simulink library "MIL_Test"  (Simulink 6.6)
undefined symbols (not defined in the file or in its folder): getdatatypespecs, slcm, StepSize
libraries: simulink x71, MIL_Test x6
(part 3 of 8)

== system MIL_Test/Validation Function/Feature extraction/Complete step detection/Step detection ==
  R : Inport
  Step : Inport  Port=2
  Step response : Inport  Port=3
  Active if signals constant for some specified time : Subsystem
  Detect constant : Subsystem  TreatAsAtomicUnit=on  mask(Feature extraction block){RT=0.0001}
      mask prompts: RT "Relative tolerance in %"
      mask help: Detect if the signal value is constant (using the last two signal values) allowing for a user-defined relative deviation
      mask CallbackString:
      | if or( (str2double(get_param(gcb,'RT')) < 0), (str2double(get_param(gcb,'RT')) > 100))
      |     error(['Relative tolerance value (' get_param(gcb,'RT') ') out of range. Please give a value between 0 and 100.']);
      | else
      |     set_param([gcb '/Relative tolerance/Relative Tolerance'],'Value',get_param(gcb,'RT'));
      | end
  Detect decrease : Subsystem  TreatAsAtomicUnit=on  mask(Detect increase){Param=0}
      mask prompts: Param "Mask Parameter 1:"
  Detect increase : Subsystem  TreatAsAtomicUnit=on  mask(Detect increase){Param=0}
      mask prompts: Param "Mask Parameter 1:"
  Detect increase2 : Subsystem  TreatAsAtomicUnit=on  mask(Detect increase){Param=0}
      mask prompts: Param "Mask Parameter 1:"
  Hold1 : Subsystem  TreatAsAtomicUnit=on
      mask Display: patch(-0.31+[0.4 0.46 0.46 0.54 0.54 0.6 0.6 0.55 0.55 0.45 0.45 0.4],-0.19+[0.85 0.85 0.95 0.95 0.85 0.85 0.87 0.87 0.96 0.96 0.87 0.87],[0 0 0]);
  Logical Operator : Logic  AllPortsSameDT=off  OutDataTypeMode=Boolean
  Logical Operator1 : Logic  Operator=NOT  AllPortsSameDT=off  OutDataTypeMode=Boolean
  Logical Operator2 : Logic  Operator=OR  Inputs=3  AllPortsSameDT=off  OutDataTypeMode=Boolean
  Memory2 : Memory
  End of complete step : Outport
  wires:
  Detect increase/1(Increase) -> Logical Operator2/1
  Detect constant/1(Constant) -> Logical Operator1/1
  Detect decrease/1(Decrease) -> Logical Operator2/2
  Logical Operator2/1 -> Hold1/1(" ")
  R/1 -> Hold1/2("    ")
  Step/1 -> Active if signals constant for some specified time/1(Signal1), Detect constant/1(Signal)
  Step response/1 -> Active if signals constant for some specified time/2(Signal 2)
  Active if signals constant for some specified time/1(Constant signals) -> Detect decrease/1(Signal), Detect increase/1(Signal), Detect increase2/1(Signal)
  Hold1/1("  ") -> Memory2/1
  Logical Operator/1 -> End of complete step/1
  Memory2/1 -> Logical Operator/2
  Detect increase2/1(Increase) -> Logical Operator/1
  Logical Operator1/1 -> Logical Operator2/3

== system MIL_Test/Validation Function/Feature extraction/Complete step detection/Step detection reset ==
  Step : Inport
  Step response : Inport  Port=2
  Active if signals constant for some specified time : Subsystem
  Logical Operator : Logic  AllPortsSameDT=off  OutDataTypeMode=Boolean
  Memory : Memory
  Step detection : Subsystem  TreatAsAtomicUnit=on  mask(Feature extraction block){StepSize=10}
      mask prompts: StepSize "Minimum step size"
      mask help: Detect a step in the signal. The minimum step size is defined by the user.
      mask CallbackString:
      | if str2double(get_param(gcb,'StepSize')) <= 0
      |     error(['Minimum step size (' get_param(gcb,'StepSize') ') out of range. Please give a value greater than zero.']);
      | else
      |     set_param([gcb '/Min step size'],'Value',get_param(gcb,'StepSize'));
      | end
  R : Outport
  wires:
  Logical Operator/1 -> R/1
  Step detection/1(Step) -> Logical Operator/2
  Step response/1 -> Active if signals constant for some specified time/1(Signal1)
  Memory/1 -> Logical Operator/1
  Active if signals constant for some specified time/1(Constant signals) -> Memory/1
  Step/1 -> Active if signals constant for some specified time/2(Signal 2), Step detection/1(Signal)

== system MIL_Test/Validation Function/Feature extraction/Detect constant/Relative tolerance ==
  sig : Inport
  ref : Inport  Port=2
  Abs : Abs
  Abs1 : Abs
  Add : Sum  Inputs=+-  OutScaling=2^-10
  Divide1 : Product  Inputs=**/  OutScaling=2^-10
  Max : Constant  Value=100
  Relational Operator : RelationalOperator  Operator===  LogicOutDataTypeMode=Boolean
  Relative Tolerance : Constant
  sig == ref : Outport
  wires:
  Abs1/1 -> Divide1/1
  Relational Operator/1 -> sig == ref/1
  Relative Tolerance/1 -> Divide1/2
  Max/1 -> Divide1/3
  Divide1/1 -> Relational Operator/2
  ref/1 -> Abs1/1, Add/2
  sig/1 -> Add/1
  Add/1 -> Abs/1
  Abs/1 -> Relational Operator/1

== system MIL_Test/Validation Function/Feature extraction/Linear relation/Relative tolerance ==
  sig : Inport
  ref : Inport  Port=2
  Abs : Abs
  Abs1 : Abs
  Add : Sum  Inputs=+-  OutScaling=2^-10
  Divide1 : Product  Inputs=**/  OutScaling=2^-10
  Max : Constant  Value=100
  Relational Operator : RelationalOperator  Operator=<=  LogicOutDataTypeMode=Boolean
  Relative Tolerance : Constant  Value=0.0001
  sig == ref : Outport
  wires:
  Abs1/1 -> Divide1/1
  Relational Operator/1 -> sig == ref/1
  Relative Tolerance/1 -> Divide1/2
  Max/1 -> Divide1/3
  Divide1/1 -> Relational Operator/2
  ref/1 -> Abs1/1, Add/2
  sig/1 -> Add/1
  Add/1 -> Abs/1
  Abs/1 -> Relational Operator/1

== system MIL_Test/Validation Function/Feature extraction/Signal value @ maximum/Local maximum ==
  Signal : Inport
  Clock : Clock
      settings: Decimation=10
  Clock1 : Clock
      settings: Decimation=10
  Logical Operator : Logic  AllPortsSameDT=off  OutDataTypeMode=Boolean
  Memory : Memory
  Memory1 : Memory
  Relational Operator : RelationalOperator  Operator=<  LogicOutDataTypeMode=Boolean
  Relational Operator1 : RelationalOperator  Operator=>  LogicOutDataTypeMode=Boolean
  Switch : Switch  Criteria=u2 > Threshold
  Switch1 : Switch  Criteria=u2 > Threshold
  Maximum : Outport
  wires:
  Switch1/1 -> Relational Operator1/2
  Memory1/1 -> Switch1/1
  Clock1/1 -> Switch1/2
  Switch/1 -> Relational Operator1/1, Switch1/3, Memory1/1, Relational Operator/2
  Memory/1 -> Switch/1
  Clock/1 -> Switch/2
  Relational Operator/1 -> Logical Operator/1
  Relational Operator1/1 -> Logical Operator/2
  Logical Operator/1 -> Maximum/1
  Signal/1 -> Switch/3, Memory/1, Relational Operator/1

== system MIL_Test/Validation Function/Feature extraction/Step response characteristics/Step response characteristics extraction ==
  R : Inport
  Step : Inport  Port=2
  Step response : Inport  Port=3
  Clock : Clock
      settings: Decimation=10
  Expected set point and step parameters : Subsystem  TreatAsAtomicUnit=on
  Extract maximum overshoot : Subsystem
  Extract rise time : Subsystem
  Extract settling time : Subsystem
  Extract steady state error : Subsystem
  Memory : Memory
  Static Gain : Constant  Value=0.8333
  Step time : Subsystem  TreatAsAtomicUnit=on
  Rise time : Outport  DataType=double
  Maximum overshoot : Outport  Port=2  DataType=double
  Settling time : Outport  Port=3  DataType=double
  Steady state error : Outport  Port=4  DataType=double
  wires:
  Expected set point and step parameters/1(Step sign) -> Extract maximum overshoot/3(Step sign)
  Expected set point and step parameters/3(Response step size) -> Extract rise time/4(Response step size)
  Step response/1 -> Extract rise time/1(Step response), Extract maximum overshoot/1(Step response), Extract settling time/1(Step response), Extract steady state error/1(Step response)
  Step time/1(Time) -> Extract settling time/4(Step time)
  Expected set point and step parameters/2(Set point) -> Extract rise time/3(Set point), Extract settling time/2(Set point), Extract steady state error/2(Set point)
  Extract steady state error/1(ss error) -> Steady state error/1
  Memory/1 -> Expected set point and step parameters/1(Step/z)
  Clock/1 -> Step time/1(Clock)
  Step/1 -> Expected set point and step parameters/2(Step), Memory/1
  R/1 -> Extract settling time/3(Reset), Extract maximum overshoot/2(Reset), Extract rise time/2(Reset), Expected set point and step parameters/Trigger, Step time/Trigger
  Static Gain/1 -> Expected set point and step parameters/3(Static Gain)
  Extract settling time/1(Settling time) -> Settling time/1
  Extract maximum overshoot/1(Maximum overshoot) -> Maximum overshoot/1
  Extract rise time/1(Rise time) -> Rise time/1

== system MIL_Test/Validation Function/Feature extraction/Step response characteristics/Step response reset ==
  Step : Inport
  Step response : Inport  Port=2
  Active if signals constant for some specified time : Subsystem
  Logical Operator : Logic  AllPortsSameDT=off  OutDataTypeMode=Boolean
  Memory : Memory
  Step detection : Subsystem  TreatAsAtomicUnit=on  mask(Feature extraction block){StepSize=1}
      mask prompts: StepSize "Minimum step size"
      mask help: Detect a step in the signal. The minimum step size is defined by the user.
      mask CallbackString:
      | if str2double(get_param(gcb,'StepSize')) <= 0
      |     error(['Minimum step size (' get_param(gcb,'StepSize') ') out of range. Please give a value greater than zero.']);
      | else
      |     set_param([gcb '/Min step size'],'Value',get_param(gcb,'StepSize'));
      | end
  R : Outport
  wires:
  Logical Operator/1 -> R/1
  Step detection/1(Step) -> Logical Operator/2
  Step response/1 -> Active if signals constant for some specified time/1(Signal1)
  Memory/1 -> Logical Operator/1
  Active if signals constant for some specified time/1(Constant signals) -> Memory/1
  Step/1 -> Active if signals constant for some specified time/2(Signal 2), Step detection/1(Signal)

== system MIL_Test/Validation Function/Feature extraction/Step response characteristics/Step response trigger ==
  Steady state error : Inport
  Step response : Inport  Port=2
  Abs : Abs
  Active if signals constant for some specified time : Subsystem
  Compare To Constant : Subsystem  mask(Compare To Constant){relop=<=, const=0.5, LogicOutDataTypeMode=uint8, ZeroCross=off}
      mask prompts: relop "Operator:"; const "Constant value:"; LogicOutDataTypeMode "Output data type mode:"; ZeroCross "Enable zero crossing detection"
      mask help: Determine how a signal compares to a constant.
      mask init:
      | blkName = gcb;
      | 
      | if strcmp(get_param(gcbh,'LogicOutDataTypeMode'),'boolean')
      | 	setValue = 'Boolean';
      | else
      | 	setValue = 'Specify via dialog';
      | end
      | 
      | set_param([blkName,'/Compare'],'relop',relop, ...
      | 	'LogicOutDataTypeMode', setValue, 'ZeroCross', ZeroCross);
      | 
      | if length(const) == 1
      |  str = [relop,' ',num2str(double(const))];
      | else
      |   str = [relop,' C'];
      | end
      mask StyleString: popup(==|~=|<|<=|>=|>),edit,popup(uint8|boolean),checkbox
      mask Display: disp(str)
  Data Type Conversion : DataTypeConversion
  Data Type Conversion1 : DataTypeConversion
  Detect increase : Subsystem  TreatAsAtomicUnit=on
  Logical Operator : Logic  AllPortsSameDT=off  OutDataTypeMode=Boolean  LogicDataType=double
  Rise time T : Outport  DataType=double
  Overshoot T : Outport  Port=2  DataType=double
  Settling time T : Outport  Port=3  DataType=double
  Steady state error T : Outport  Port=4  DataType=double
  wires:
  Logical Operator/1 -> Data Type Conversion/1
  Detect increase/1(Increase) -> Data Type Conversion1/1, Logical Operator/2
  Abs/1 -> Compare To Constant/1(u)
  Compare To Constant/1(y) -> Logical Operator/1
  Steady state error/1 -> Abs/1
  Step response/1 -> Active if signals constant for some specified time/1(Signal1), Active if signals constant for some specified time/2(Signal 2)
  Active if signals constant for some specified time/1(Constant signals) -> Detect increase/1(Signal)
  Data Type Conversion1/1 -> Steady state error T/1
  Data Type Conversion/1 -> Settling time T/1, Overshoot T/1, Rise time T/1

== system MIL_Test/Validation Function/Feature extraction/Time @ sig = x/Relative tolerance ==
  sig : Inport
  ref : Inport  Port=2
  Abs : Abs
  Abs1 : Abs
  Add : Sum  Inputs=+-  OutScaling=2^-10
  Divide1 : Product  Inputs=**/  OutScaling=2^-10
  Max : Constant  Value=100
  Relational Operator : RelationalOperator  Operator=<=  LogicOutDataTypeMode=Boolean
  Relative Tolerance : Constant  Value=0.0001
  sig == ref : Outport
  wires:
  Abs1/1 -> Divide1/1
  Relational Operator/1 -> sig == ref/1
  Relative Tolerance/1 -> Divide1/2
  Max/1 -> Divide1/3
  Divide1/1 -> Relational Operator/2
  ref/1 -> Abs1/1, Add/2
  sig/1 -> Add/1
  Add/1 -> Abs/1
  Abs/1 -> Relational Operator/1

== system MIL_Test/Validation Function/Feature extraction/Time since signal constant/Detect constant ==
  Signal : Inport
  Clock : Clock
      settings: Decimation=10
  Constant1 : Constant  Value=0  OutDataTypeMode=boolean
  Memory : Memory
  Relative tolerance : Subsystem
  Switch : Switch  Criteria=u2 > Threshold
  Constant : Outport
  wires:
  Switch/1 -> Constant/1
  Relative tolerance/1(sig == ref) -> Switch/1
  Clock/1 -> Switch/2
  Constant1/1 -> Switch/3
  Memory/1 -> Relative tolerance/2(ref)
  Signal/1 -> Relative tolerance/1(sig), Memory/1

== system MIL_Test/Validation Function/TODO/<system name>/<Requirement name> ==
  InOut Bus : Inport
  <Assertions name> : Subsystem  Description=Assertions template. Create a new assertions block from this template.
  <Preconditions name> : Subsystem  Description=Preconditions template. Create new preconditions blocks using this template.
  Bus Creator : BusCreator  Inputs=1
  Test Info : Outport
  wires:
  <Preconditions name>/1(Activate) -> <Assertions name>/1(Precond)
  Bus Creator/1 -> Test Info/1
  <Assertions name>/1(VF info) -> Bus Creator/1
  InOut Bus/1 -> <Preconditions name>/1(InOut Bus), <Assertions name>/2(InOut Bus)

== system MIL_Test/Validation Function/TODO/Assertions/Fault info ==
  Local Verdict : Inport
  Expected lower limit : Inport  Port=2
  Expected upper limit : Inport  Port=3
  Actual Data : Inport  Port=4
  Enable : EnablePort
  Assertions : Constant  Value=Ass
  Bus Creator : BusCreator  Inputs=5
  Bus Creator1 : BusCreator  Inputs=3
  Data Type Conversion{,1..3} (4 alike) : DataTypeConversion
  Preconditions : Constant  Value=Pre
  Requirement : Constant  Value=Req
  VF info : Outport  OutputWhenDisabled=reset  InitialOutput=[2]
  wires:
  Requirement/1 -> Bus Creator1/3  "Requirement"
  Preconditions/1 -> Bus Creator1/2  "Preconditions"
  Assertions/1 -> Bus Creator1/1  "Assertions"
  Data Type Conversion3/1 -> Bus Creator/4  "Actual data"
  Data Type Conversion2/1 -> Bus Creator/3  "Expected upper limit"
  Data Type Conversion1/1 -> Bus Creator/2  "Expected lower limit"
  Data Type Conversion/1 -> Bus Creator/1  "Local verdict"
  Local Verdict/1 -> Data Type Conversion/1  "Local verdict"
  Expected upper limit/1 -> Data Type Conversion2/1  "Expected upper limit"
  Expected lower limit/1 -> Data Type Conversion1/1  "Expected lower limit"
  Actual Data/1 -> Data Type Conversion3/1  "Actual Data"
  Bus Creator1/1 -> Bus Creator/5  "Source"
  Bus Creator/1 -> VF info/1

== system MIL_Test/Validation Function/TODO/Assertions/Signal comparison ==
  Bound : Subsystem  mask(Bound){cm=>=, Lower=0, Upper=1}
      mask prompts: cm "Comparison method:"; Upper "Mask Parameter 3:"
      mask help:
      | Compare a signal with a reference using the specified comparison method.
      |
      | Output verdict V and lower (LL) and upper (UL) limits for reporting.
      |
      | For '==' or '~=' use "Range - Gap"
      mask init:
      | set_param([get_param(gcb,'Parent') '/' get_param(gcb,'Name') '/Relational Operator'],'Operator',get_param(gcb,'cm'));
      | set_param(gcb,'Upper',num2str(uint8(max(get_param([get_param(gcb,'Parent') '/' get_param(gcb,'Name') '/Relational Operator'],'Operator') == '>'))));
      | set_param(gcb,'Lower',num2str(uint8(max(get_param([get_param(gcb,'Parent') '/' get_param(gcb,'Name') '/Relational Operator'],'Operator') == '<'))));
      mask StyleString: popup(>|>=|<=|<),edit,edit
      mask Display:
      | port_label('output', 1, 'V');
      | port_label('output', 2, 'LL');
      | port_label('output', 3, 'UL');
      | port_label('input', 1, 'Sig');
      | port_label('input', 2, 'Ref');
      | text(0.05,0.5,get_param(get_param([get_param(gcb,'Parent') '/' get_param(gcb,'Name') '/Relational Operator'],'handle'),'Operator'));
  Range - Gap Absolute tolerance : Subsystem  mask(Range - Gap Absolute Tolerance){GorR=Range, AbsoluteTolerance=100}
      mask prompts: GorR "Use range or gap"; AbsoluteTolerance "Absolute Tolerance"
      mask help:
      | Check that a signal stays inside a range or outside a gap around a reference signal. Specify the range or the gap absolute to the reference signal.
      |
      | Output verdict V and lower (LL) and upper (UL) limits for reporting.
      mask init: same as MIL_Test/Test Data/Signal comparison/Range - Gap Relative tolerance Precond
      mask StyleString: popup(Range|Gap  ),edit
      mask Display:
      | port_label('output',1,'V');
      | port_label('output',2,'LL');
      | port_label('output',3,'UL');
      | port_label('input',1,'Sig');
      | port_label('input',2,'Ref');
      | text(0.40,0.53,'+');
      | text(0.415,0.46,'-');
      | text(0.5,0.5,num2str(AbsoluteTolerance));
      | text(0.05,0.5,helpVariable2);
  Range - Gap Relative tolerance : Subsystem  mask(Range - Gap Relative Tolerance){GorR=Range, RelativeTolerance=1}
      mask prompts: GorR "Use range or gap"; RelativeTolerance "Relative Tolerance in Percent"
      mask help:
      | Check that a signal stays inside a range or outside a gap around a reference signal. Specify the range or the gap relative to the reference signal.
      |
      | Output verdict V and lower (LL) and upper (UL) limits for reporting.
      mask init: same as MIL_Test/Test Data/Signal comparison/Range - Gap Relative tolerance Precond
      mask StyleString: popup(Range|Gap  ),edit
      mask Display:
      | port_label('output',1,'V');
      | port_label('output',2,'LL');
      | port_label('output',3,'UL');
      | port_label('input',1,'Sig');
      | port_label('input',2,'Ref');
      | text(0.425,0.5,[num2str(RelativeTolerance) ' %']);
      | text(0.05,0.5,helpVariable2);
  Range - Gap Tolerance range : Subsystem  mask(Range - Gap Tolerance range){GorR=Range}
      mask prompts: GorR "Use range or gap"
      mask help:
      | Check that a signal stays inside a dynamically specified value range.
      |
      | Output verdict V and lower (LL) and upper (UL) limits for reporting.
      mask init:
      | if max(get_param(gcb,'GorR') == ' ') % Gap
      |     helpVariable1 = '<=';
      | else % Range
      |     helpVariable1 = '>=';
      | end
      | set_param([get_param(gcb,'Parent') '/' get_param(gcb,'Name') '/Relational Operator'],'Operator',helpVariable1);
      | clear helpVariable1;
      mask StyleString: popup(Range|Gap  )
      mask Display:
      | port_label('output',1,'V');
      | port_label('output',2,'LL');
      | port_label('output',3,'UL');
      | port_label('input',1,'Sig');
      | port_label('input',2,'Lower Bound');
      | port_label('input',3,'Upper Bound');
      | patch(0.05+[0.3 0.7 0.7 0.3],-0.05+[0.8 0.8 0.9 0.9],[1 1 1]*double(not(max(get_param(gcb,'GorR') == ' '))));
      | patch(0.05+[0.3 0.7 0.7 0.3],-0.05+[0.9 0.9 0.95 0.95],[1 1 1]*double(max(get_param(gcb,'GorR') == ' ')));
      | patch(0.05+[0.3 0.7 0.7 0.3],-0.05+[0.75 0.75 0.8 0.8],[1 1 1]*double(max(get_param(gcb,'GorR') == ' ')));
      | patch(0.05+[0.25 0.25 0.8 0.8 0.26 0.26],[0.95 0.65 0.65 0.66 0.66 0.95],[0 0 0]);
      | patch(0.033+[0.27 0.22 0.23 0.27 0.31 0.32 0.27],0.02+[0.95 0.85 0.85 0.89 0.85 0.85 0.95],[0 0 0]);
      | patch(0.17+[0.7 0.6 0.6 0.65 0.6 0.6 0.7],-0.043+[0.7 0.63 0.64 0.7 0.76 0.77 0.7],[0 0 0]);

== system MIL_Test/Validation Function/TODO/Model Info/EmptySubsystem ==

== system MIL_Test/Validation Function/TODO/Preconditions/Signal comparison ==
  Bound : Subsystem  mask(Bound){cm=>=}
      mask prompts: cm "Comparison method:"
      mask help:
      | Compare a signal with a reference using the specified comparison method.
      |
      | For '==' or '~=' use "Range - Gap"
      mask init:
      | bp = get_param(gcbh,'Parent');
      | bn = get_param(gcbh,'Name');
      | set_param([bp '/' bn '/RelOp'],'Operator',get_param(gcbh,'cm'));
      mask StyleString: popup(>|>=|<=|<)
      mask Display:
      | port_label('output', 1, 'A');
      | port_label('input', 1, 'Sig');
      | port_label('input', 2, 'Ref');
      | text(0.05,0.5,get_param(get_param([get_param(gcb,'Parent') '/' get_param(gcb,'Name') '/RelOp'],'handle'),'Operator'));
  Range - Gap Absolute tolerance : Subsystem  mask(Range - Gap Absolute Tolerance){GorR=Range, AbsoluteTolerance=100}
      mask prompts: GorR "Use range or gap"; AbsoluteTolerance "Absolute Tolerance"
      mask help: Check that a signal stays inside a range or outside a gap around a reference signal. Specify the range or the gap absolute to the reference signal.
      mask init:
      | if max(get_param(gcb,'GorR') == ' ') % Gap
      |     helpVariable1 = '>=';
      |     helpVariable2 = '~=';
      | else % Range
      |     helpVariable1 = '<=';
      |     helpVariable2 = '==';
      | end
      | set_param([get_param(gcb,'Parent') '/' get_param(gcb,'Name') '/Relational Operator'],'Operator',helpVariable1);
      | set_param(gcb,'Op',helpVariable2);
      | clear helpVariable1;
      mask StyleString: popup(Range|Gap  ),edit
      mask Display:
      | port_label('output',1,'A');
      | port_label('input',1,'Sig');
      | port_label('input',2,'Ref');
      | text(0.40,0.53,'+');
      | text(0.415,0.46,'-');
      | text(0.5,0.5,num2str(AbsoluteTolerance));
      | text(0.05,0.5,helpVariable2);
  Range - Gap Relative tolerance : Subsystem  mask(Range - Gap Relative Tolerance){GorR=Range, RelativeTolerance=1}
      mask prompts: GorR "Use range or gap"; RelativeTolerance "Relative Tolerance in Percent"
      mask help: Check that a signal stays inside a range or outside a gap around a reference signal. Specify the range or the gap relative to the reference signal.
      mask init: same as MIL_Test/Test Data/Signal comparison/Range - Gap Relative tolerance Precond
      mask StyleString: popup(Range|Gap  ),edit
      mask Display:
      | port_label('output',1,'A');
      | port_label('input',1,'Sig');
      | port_label('input',2,'Ref');
      | text(0.425,0.5,[num2str(RelativeTolerance) ' %']);
      | text(0.05,0.5,helpVariable2);
  Range - Gap Tolerance range : Subsystem  mask(Range - Gap Tolerance range){GorR=Range}
      mask prompts: GorR "Use range or gap"
      mask help: Check that a signal stays inside a dynamically specified value range.
      mask init: same as MIL_Test/Validation Function/TODO/Assertions/Signal comparison/Range - Gap Tolerance range
      mask StyleString: popup(Range|Gap  )
      mask Display:
      | port_label('output',1,'A');
      | port_label('input',1,'Sig');
      | port_label('input',2,'Lower Bound');
      | port_label('input',3,'Upper Bound');
      | patch(0.05+[0.3 0.7 0.7 0.3],-0.05+[0.8 0.8 0.9 0.9],[1 1 1]*double(not(max(get_param(gcb,'GorR') == ' '))));
      | patch(0.05+[0.3 0.7 0.7 0.3],-0.05+[0.9 0.9 0.95 0.95],[1 1 1]*double(max(get_param(gcb,'GorR') == ' ')));
      | patch(0.05+[0.3 0.7 0.7 0.3],-0.05+[0.75 0.75 0.8 0.8],[1 1 1]*double(max(get_param(gcb,'GorR') == ' ')));
      | patch(0.05+[0.25 0.25 0.8 0.8 0.26 0.26],[0.95 0.65 0.65 0.66 0.66 0.95],[0 0 0]);
      | patch(0.033+[0.27 0.22 0.23 0.27 0.31 0.32 0.27],0.02+[0.95 0.85 0.85 0.89 0.85 0.85 0.95],[0 0 0]);
      | patch(0.17+[0.7 0.6 0.6 0.65 0.6 0.6 0.7],-0.043+[0.7 0.63 0.64 0.7 0.76 0.77 0.7],[0 0 0]);

== system MIL_Test/Validation Function/TODO/Validation FunctionsTemplate/Arbitration ==
  In1 : Inport
  Collect Verdicts : MinMax  Inputs=3
  Memory : Memory  Orientation=left  X0=2
  Out1 : Outport
  wires:
  Collect Verdicts/1 -> Memory/1, Out1/1
  In1/1 -> Collect Verdicts/1
  Memory/1 -> Collect Verdicts/3

== system MIL_Test/Validation Function/TODO/Validation FunctionsTemplate/Datatype conversion ==
  InOutBus : Inport
  Bus Creator{,1..5} (6 alike) : BusCreator  Inputs=2
  Bus Selector : BusSelector  OutputSignals=Inputs,Outputs
  Bus Selector1 : BusSelector  OutputSignals=v_Fzg,signal2
  Bus Selector2 : BusSelector  OutputSignals=signal1,signal2
  Bus Selector3 : BusSelector  OutputSignals=phi_Acc,phi_Brake
  Bus Selector4 : BusSelector  OutputSignals=T_des_Drive,T_des_Brake
  Bus Selector5 : BusSelector  OutputSignals=AccPedal,BrakePedal
  Data Type Conversion{,1..6} (7 alike) : DataTypeConversion
  InOut Bus : Outport
  wires:
  Bus Creator5/1 -> InOut Bus/1  "InOutBus"
  Bus Creator4/1 -> Bus Creator5/2  "Outputs"
  Bus Creator3/1 -> Bus Creator5/1  "Inputs"
  Bus Creator1/1 -> Bus Creator4/2
  Bus Creator/1 -> Bus Creator4/1
  Data Type Conversion/1 -> Bus Creator3/1  "v_Fzg"
  Bus Creator2/1 -> Bus Creator3/2  "signal2"
  Data Type Conversion2/1 -> Bus Creator2/2  "phi_Brake"
  Data Type Conversion1/1 -> Bus Creator2/1  "phi_Acc"
  Data Type Conversion6/1 -> Bus Creator1/2  "BrakePedal"
  Data Type Conversion5/1 -> Bus Creator1/1  "AccPedal"
  Data Type Conversion4/1 -> Bus Creator/2  "T_des_Brake"
  Data Type Conversion3/1 -> Bus Creator/1  "T_des_Drive"
  Bus Selector5/2 -> Data Type Conversion6/1  "<BrakePedal>"
  Bus Selector5/1 -> Data Type Conversion5/1  "<AccPedal>"
  Bus Selector4/2 -> Data Type Conversion4/1  "<T_des_Brake>"
  Bus Selector4/1 -> Data Type Conversion3/1  "<T_des_Drive>"
  Bus Selector3/2 -> Data Type Conversion2/1  "<phi_Brake>"
  Bus Selector3/1 -> Data Type Conversion1/1  "<phi_Acc>"
  Bus Selector1/1 -> Data Type Conversion/1  "<v_Fzg>"
  Bus Selector2/2 -> Bus Selector5/1  "<signal2>"
  Bus Selector2/1 -> Bus Selector4/1  "<signal1>"
  Bus Selector1/2 -> Bus Selector3/1  "<signal2>"
  Bus Selector/2 -> Bus Selector2/1  "<Outputs>"
  Bus Selector/1 -> Bus Selector1/1  "<Inputs>"
  InOutBus/1 -> Bus Selector/1

== system MIL_Test/Validation Function/TODO/Validation FunctionsTemplate/Requirement ==
  InOut Bus : Inport
  Assertions : Subsystem  TreatAsAtomicUnit=on
  Bus Creator : BusCreator  Inputs=1
  Preconditions : Subsystem
  Validation Information : Outport
  wires:
  Assertions/1(VF info) -> Bus Creator/1
  Bus Creator/1 -> Validation Information/1
  InOut Bus/1 -> Preconditions/1(InOut Bus), Assertions/2(InOut Bus)
  Preconditions/1(Activate) -> Assertions/1(Activate)

== system MIL_Test/Validation Function/TODO/Validation FunctionsTemplate/Requirement2 ==
  InOut Bus : Inport
  Assertions : Subsystem  TreatAsAtomicUnit=on
  Bus Creator : BusCreator  Inputs=1
  Preconditions : Subsystem
  Validation Information : Outport
  wires:
  Preconditions/1(Activate) -> Assertions/1(Activate)
  InOut Bus/1 -> Assertions/2(InOut Bus), Preconditions/1(InOut Bus)
  Bus Creator/1 -> Validation Information/1
  Assertions/1(VF info) -> Bus Creator/1

== system MIL_Test/Validation Function/Test Evaluation Architecture/<system name>/<Requirement name> ==
  InOut Bus : Inport
  <Assertions name> : Subsystem  Description=Assertions template. Create a new assertions block from this template.
  <Preconditions name> : Subsystem  Description=Preconditions template. Create new preconditions blocks using this template.
  Bus Creator : BusCreator  Inputs=1
  Test Info : Outport
  wires:
  InOut Bus/1 -> <Assertions name>/2(InOut Bus), <Preconditions name>/1(InOut Bus)
  <Assertions name>/1(VF info) -> Bus Creator/1
  Bus Creator/1 -> Test Info/1
  <Preconditions name>/1(Activate) -> <Assertions name>/1(Precond)

== system MIL_Test/Validation Function/Test Evaluation Architecture/<system name>/Arbitration ==
  In1 : Inport
  Collect Verdicts : MinMax  Inputs=2
  Memory : Memory  Orientation=left  X0=2
  Out1 : Outport
  wires:
  Memory/1 -> Collect Verdicts/2
  Collect Verdicts/1 -> Memory/1, Out1/1
  In1/1 -> Collect Verdicts/1

== system MIL_Test/Test Control/Test Control Architecture/Connection Helpers/TestControl for  TestCases Sequencing NoMask/IF Signal@SimStopTime for TC = value1 ==
  Signal : Inport
  Current Sim StopTime : Constant  Value=currentStopTime
  If : If  IfExpression=u1 ~= 1
  Model Info : simulink/Model-Wide Utilities/Model Info  SystemSampleTime=-1  InitialBlockCM=None  BlockCM=None  Frame=on  DisplayStringWithTags=|  HorizontalTextAlignment=Center  LeftAlignmentValue=0.5  SourceBlockDiagram=MIL_Test  TagMaxNumber=20
      | Flag Fullfillment = 1, then condition is true 
      | Flag Fullfillment = 0, then condition is false
  if Signal@t for TC = pass : Subsystem
  "if false, then  TC4 for 200" : Subsystem
  "if true, then  TC2 for 400" : Subsystem
  Fulfillment : Outport
  wires:
  Current Sim StopTime/1 -> if Signal@t for TC = pass/1(@time)
  Signal/1 -> if Signal@t for TC = pass/2(Signal1)
  If/1 -> "if false, then  TC4 for 200"/Action
  If/2 -> "if true, then  TC2 for 400"/Action
  if Signal@t for TC = pass/1(Control Seq1) -> Fulfillment/1

== system MIL_Test/Test Control/Test Control Architecture/Connection Helpers/TestControl for  TestCases Sequencing NoMask/IF signal @[timeUp, timeDown] for TC = value1 ==
  Signal : Inport
  TimeDown : Constant  Value=timeDown
  TimeUp : Constant  Value=timeUp
  if Signal@ [TDown,TUp]  for TC = Value : Subsystem
  Fulfillment : Outport
  wires:
  TimeDown/1 -> if Signal@ [TDown,TUp]  for TC = Value/1(@timeDown)
  TimeUp/1 -> if Signal@ [TDown,TUp]  for TC = Value/2(@timeUp)
  Signal/1 -> if Signal@ [TDown,TUp]  for TC = Value/3(Signal)
  if Signal@ [TDown,TUp]  for TC = Value/1(Control Seq) -> Fulfillment/1

== system MIL_Test/Test Control/Test Control Architecture/Connection Helpers/TestControl for  TestCases Sequencing NoMask/IF signal@time for TC = value1 ==
  Signal : Inport
  given Time : Constant  Value=time
  if Signal@t for TC = pass : Subsystem
  Fulfillment : Outport
  wires:
  given Time/1 -> if Signal@t for TC = pass/1(@time)
  Signal/1 -> if Signal@t for TC = pass/2(Signal1)
  if Signal@t for TC = pass/1(Control Seq) -> Fulfillment/1

== system MIL_Test/Test Control/Test Control Architecture/Test Control Conditions/IF Signal@SimStopTime for TC = value1/if Signal@t for TC = pass ==
  @time : Inport
  Signal1 : Inport  Port=2
  ClockAtEnd : Clock
      settings: Decimation=10
  Relational Operator1 : RelationalOperator  LogicOutDataTypeMode=Boolean
  check in range : Subsystem  TreatAsAtomicUnit=on
  Control Seq1 : Outport
  wires:
  Relational Operator1/1 -> check in range/Enable, check in range/1(@[time])
  check in range/1(Control Seq) -> Control Seq1/1
  Signal1/1 -> check in range/2(Signal)
  @time/1 -> Relational Operator1/2
  ClockAtEnd/1 -> Relational Operator1/1

== system MIL_Test/Test Control/Test Control Architecture/Test Control Conditions/IF Signal@SimStopTime for TC = value1/if false, then  TC4 for 200 ==
  Action Port : ActionPort
  Embedded MATLAB Function : Stateflow chart

== system MIL_Test/Test Control/Test Control Architecture/Test Control Conditions/IF Signal@SimStopTime for TC = value1/if true, then  TC2 for 400 ==
  Action Port : ActionPort
  Embedded MATLAB Function : Stateflow chart

== system MIL_Test/Test Control/Test Control Architecture/Test Control Conditions/IF signal @[timeUp, timeDown] for TC = value1/if Signal@ [TDown,TUp]  for TC = Value ==
  @timeDown : Inport
  @timeUp : Inport  Port=2
  Signal : Inport  Port=3
  ClockDuring : Clock
      settings: Decimation=10
  Logical Operator1 : Logic  AllPortsSameDT=off  OutDataTypeMode=Boolean
  Relational Operator1 : RelationalOperator  LogicOutDataTypeMode=Boolean
  Relational Operator2 : RelationalOperator  Operator=<=  LogicOutDataTypeMode=Boolean
  check in range : Subsystem  TreatAsAtomicUnit=on
  Control Seq : Outport
  wires:
  check in range/1(Control Seq) -> Control Seq/1
  Signal/1 -> check in range/2(Signal)
  Logical Operator1/1 -> check in range/Enable, check in range/1(@[time])
  Relational Operator2/1 -> Logical Operator1/2
  Relational Operator1/1 -> Logical Operator1/1
  @timeUp/1 -> Relational Operator2/2
  @timeDown/1 -> Relational Operator1/2
  ClockDuring/1 -> Relational Operator2/1, Relational Operator1/1

== system MIL_Test/Test Control/Test Control Architecture/Test Control Conditions/IF signal@time for TC = value1/if Signal@t for TC = pass ==
  @time : Inport
  Signal1 : Inport  Port=2
  ClockAtTime : Clock
      settings: Decimation=10
  Relational Operator1 : RelationalOperator  LogicOutDataTypeMode=Boolean
  check in range : Subsystem  TreatAsAtomicUnit=on
  Control Seq : Outport
  wires:
  check in range/1(Control Seq) -> Control Seq/1
  Signal1/1 -> check in range/2(Signal)
  Relational Operator1/1 -> check in range/Enable, check in range/1(@[time])
  @time/1 -> Relational Operator1/2
  ClockAtTime/1 -> Relational Operator1/1

== system MIL_Test/Test Control/Test Control Architecture/Test Control Conditions/IF signal@time1/if Signal@t for TC = pass ==
  @time : Inport
  Signal1 : Inport  Port=2
  Clock : Clock
      settings: Decimation=10
  Relational Operator1 : RelationalOperator  LogicOutDataTypeMode=Boolean
  check in range : Subsystem  TreatAsAtomicUnit=on
  Control Seq : Outport
  wires:
  Relational Operator1/1 -> check in range/Enable, check in range/1(@[time])
  check in range/1(Control Seq) -> Control Seq/1
  Signal1/1 -> check in range/2(Signal)
  @time/1 -> Relational Operator1/2
  Clock/1 -> Relational Operator1/1

== system MIL_Test/Test Control/Test Control Architecture/Test Control Conditions/IF signal@time1/if false, then  TC4 for 200 ==
  Action Port : ActionPort
  Embedded MATLAB Function : Stateflow chart

== system MIL_Test/Test Control/Test Control Architecture/Test Control Conditions/IF signal@time1/if true, then  TC2 for 400 ==
  Action Port : ActionPort
  Embedded MATLAB Function : Stateflow chart

== system MIL_Test/Test Data/Feature generation/Generate  local maximum  with given slope/Limited Ramp Increasing/Enabled Subsystem1 ==
  In2 : Inport
  Enable : EnablePort  StatesWhenEnabling=reset
  MaxValue1 : Outport  InitialOutput=[0]
  wires:
  In2/1 -> MaxValue1/1

== system MIL_Test/Test Data/Test Data Architecture/<Test data generator>/<Requirement name>/<Preconditions name> ==
  Out Bus : Inport
  <Check> : Subsystem
  Feature generation : Subsystem  TreatAsAtomicUnit=on  mask{Param=0}
      mask prompts: Param "Mask Parameter 1:"
  Activate : Outport
  <signal1> : Outport  Port=2
  wires:
  <Check>/1(A) -> Activate/1
  Feature generation/1(<signal1>) -> <signal1>/1
  Out Bus/1 -> <Check>/1(Out Bus)

== system MIL_Test/Test Data/Test Data Architecture/<Test data generator>/<Requirement name>/Initialisation & Stabilisation ==
  <Feature generation> : Subsystem  TreatAsAtomicUnit=on  mask{Param=0}
      mask prompts: Param "Mask Parameter 1:"
  <signal1> : Outport
  wires:
  <Feature generation>/1(<signal1>) -> <signal1>/1

== system MIL_Test/Validation Function/Feature extraction/Complete step detection/Step detection/Active if signals constant for some specified time ==
  Signal1 : Inport
  Signal 2 : Inport  Port=2
  Logical Operator1 : Logic  AllPortsSameDT=off  OutDataTypeMode=Boolean
  Min Time : Constant  Value=10
  MinMax : MinMax  Inputs=2
  Relational Operator2 : RelationalOperator  Operator=<=  LogicOutDataTypeMode=Boolean
  Switch : Switch  Criteria=u2 ~= 0
  Time since signal constant : Subsystem  TreatAsAtomicUnit=on  mask(Feature extraction block){RT=0.001}
      mask prompts: RT "Relative tolerance in %"
      mask help: Detect if the signal value is constant (using the last two signal values) allowing for a user-defined relative deviation
      mask CallbackString:
      | if or( (str2double(get_param(gcb,'RT')) < 0), (str2double(get_param(gcb,'RT')) > 100))
      |     error(['Relative tolerance value (' get_param(gcb,'RT') ') out of range. Please give a value between 0 and 100.']);
      | else
      |     set_param([gcb '/Detect constant/Relative tolerance/Relative Tolerance'],'Value',get_param(gcb,'RT'));
      |     set_param([gcb '/Detect constant'],'RT',get_param(gcb,'RT'));
      | end
  Time since signal constant1 : Subsystem  TreatAsAtomicUnit=on  mask(Feature extraction block){RT=0.001}
      mask prompts: RT "Relative tolerance in %"
      mask help: Detect if the signal value is constant (using the last two signal values) allowing for a user-defined relative deviation
      mask CallbackString:
      | if or( (str2double(get_param(gcb,'RT')) < 0), (str2double(get_param(gcb,'RT')) > 100))
      |     error(['Relative tolerance value (' get_param(gcb,'RT') ') out of range. Please give a value between 0 and 100.']);
      | else
      |     set_param([gcb '/Detect constant/Relative tolerance/Relative Tolerance'],'Value',get_param(gcb,'RT'));
      |     set_param([gcb '/Detect constant'],'RT',get_param(gcb,'RT'));
      | end
  Zero : Constant  Value=0
  Constant signals : Outport
  wires:
  Zero/1 -> Switch/3
  Logical Operator1/1 -> Switch/2
  MinMax/1 -> Switch/1
  Time since signal constant1/1(Trigger) -> Logical Operator1/2
  Time since signal constant/1(Trigger) -> Logical Operator1/1
  Time since signal constant/2(Feature) -> MinMax/1
  Time since signal constant1/2(Feature) -> MinMax/2
  Switch/1 -> Relational Operator2/2
  Min Time/1 -> Relational Operator2/1
  Relational Operator2/1 -> Constant signals/1
  Signal 2/1 -> Time since signal constant1/1(Signal)
  Signal1/1 -> Time since signal constant/1(Signal)

== system MIL_Test/Validation Function/Feature extraction/Complete step detection/Step detection/Detect constant ==
  Signal : Inport
  Clock : Clock
      settings: Decimation=10
  Constant1 : Constant  Value=0  OutDataTypeMode=boolean
  Memory : Memory
  Relative tolerance : Subsystem
  Switch : Switch  Criteria=u2 > Threshold
  Constant : Outport
  wires:
  Signal/1 -> Memory/1, Relative tolerance/1(sig)
  Memory/1 -> Relative tolerance/2(ref)
  Constant1/1 -> Switch/3
  Clock/1 -> Switch/2
  Relative tolerance/1(sig == ref) -> Switch/1
  Switch/1 -> Constant/1

== system MIL_Test/Validation Function/Feature extraction/Complete step detection/Step detection/Detect decrease ==
  Signal : Inport
  Clock : Clock
      settings: Decimation=10
  Memory : Memory
  Relational Operator : RelationalOperator  Operator=<  LogicOutDataTypeMode=Specify via dialog
  Switch : Switch  Criteria=u2 > Threshold
  Decrease : Outport
  wires:
  Signal/1 -> Relational Operator/1, Memory/1, Switch/3
  Relational Operator/1 -> Decrease/1
  Clock/1 -> Switch/2
  Memory/1 -> Switch/1
  Switch/1 -> Relational Operator/2

== system MIL_Test/Validation Function/Feature extraction/Complete step detection/Step detection/Detect increase ==
  Signal : Inport
  Clock : Clock
      settings: Decimation=10
  Memory : Memory
  Relational Operator : RelationalOperator  Operator=>  LogicOutDataTypeMode=Specify via dialog
  Switch : Switch  Criteria=u2 > Threshold
  Increase : Outport
  wires:
  Switch/1 -> Relational Operator/2
  Memory/1 -> Switch/1
  Clock/1 -> Switch/2
  Relational Operator/1 -> Increase/1
  Signal/1 -> Switch/3, Memory/1, Relational Operator/1

== system MIL_Test/Validation Function/Feature extraction/Complete step detection/Step detection/Detect increase2 ==
  Signal : Inport
  Clock : Clock
      settings: Decimation=10
  Memory : Memory
  Relational Operator : RelationalOperator  Operator=>  LogicOutDataTypeMode=Specify via dialog
  Switch : Switch  Criteria=u2 > Threshold
  Increase : Outport
  wires:
  Signal/1 -> Relational Operator/1, Memory/1, Switch/3
  Relational Operator/1 -> Increase/1
  Clock/1 -> Switch/2
  Memory/1 -> Switch/1
  Switch/1 -> Relational Operator/2

== system MIL_Test/Validation Function/Feature extraction/Complete step detection/Step detection/Hold1 ==
  " " : Inport
  "    " : Inport  Port=2
  Memory : Memory  Orientation=left
  Switch : Switch  Criteria=u2 ~= 0
  "  " : Outport
  wires:
  " "/1 -> Switch/2
  "    "/1 -> Switch/1
  Switch/1 -> "  "/1, Memory/1
  Memory/1 -> Switch/3

== system MIL_Test/Validation Function/Feature extraction/Complete step detection/Step detection reset/Active if signals constant for some specified time ==
  Signal1 : Inport
  Signal 2 : Inport  Port=2
  Logical Operator1 : Logic  AllPortsSameDT=off  OutDataTypeMode=Boolean
  Min Time : Constant  Value=10
  MinMax : MinMax  Inputs=2
  Relational Operator2 : RelationalOperator  Operator=<=  LogicOutDataTypeMode=Boolean
  Switch : Switch  Criteria=u2 ~= 0
  Time since signal constant : Subsystem  TreatAsAtomicUnit=on  mask(Feature extraction block){RT=0.0001}
      mask prompts: RT "Relative tolerance in %"
      mask help: Detect if the signal value is constant (using the last two signal values) allowing for a user-defined relative deviation
      mask CallbackString:
      | if or( (str2double(get_param(gcb,'RT')) < 0), (str2double(get_param(gcb,'RT')) > 100))
      |     error(['Relative tolerance value (' get_param(gcb,'RT') ') out of range. Please give a value between 0 and 100.']);
      | else
      |     set_param([gcb '/Detect constant/Relative tolerance/Relative Tolerance'],'Value',get_param(gcb,'RT'));
      |     set_param([gcb '/Detect constant'],'RT',get_param(gcb,'RT'));
      | end
  Time since signal constant1 : Subsystem  TreatAsAtomicUnit=on  mask(Feature extraction block){RT=0.0001}
      mask prompts: RT "Relative tolerance in %"
      mask help: Detect if the signal value is constant (using the last two signal values) allowing for a user-defined relative deviation
      mask CallbackString:
      | if or( (str2double(get_param(gcb,'RT')) < 0), (str2double(get_param(gcb,'RT')) > 100))
      |     error(['Relative tolerance value (' get_param(gcb,'RT') ') out of range. Please give a value between 0 and 100.']);
      | else
      |     set_param([gcb '/Detect constant/Relative tolerance/Relative Tolerance'],'Value',get_param(gcb,'RT'));
      |     set_param([gcb '/Detect constant'],'RT',get_param(gcb,'RT'));
      | end
  Zero : Constant  Value=0
  Constant signals : Outport
  wires:
  Zero/1 -> Switch/3
  Logical Operator1/1 -> Switch/2
  MinMax/1 -> Switch/1
  Time since signal constant1/1(Trigger) -> Logical Operator1/2
  Time since signal constant/1(Trigger) -> Logical Operator1/1
  Time since signal constant/2(Feature) -> MinMax/1
  Time since signal constant1/2(Feature) -> MinMax/2
  Switch/1 -> Relational Operator2/2
  Min Time/1 -> Relational Operator2/1
  Relational Operator2/1 -> Constant signals/1
  Signal 2/1 -> Time since signal constant1/1(Signal)
  Signal1/1 -> Time since signal constant/1(Signal)

== system MIL_Test/Validation Function/Feature extraction/Complete step detection/Step detection reset/Step detection ==
  Signal : Inport
  Abs : Abs
  Add : Sum  Inputs=+-  OutScaling=2^-10
  Clock : Clock
      settings: Decimation=10
  Memory : Memory
  Min step size : Constant  Value=10
  Relational Operator : RelationalOperator  LogicOutDataTypeMode=Boolean
  Switch : Switch  Criteria=u2 > Threshold
  Step : Outport
  wires:
  Switch/1 -> Add/2
  Memory/1 -> Switch/1
  Clock/1 -> Switch/2
  Signal/1 -> Add/1, Switch/3, Memory/1
  Abs/1 -> Relational Operator/1
  Min step size/1 -> Relational Operator/2
  Relational Operator/1 -> Step/1
  Add/1 -> Abs/1

== system MIL_Test/Validation Function/Feature extraction/Step response characteristics/Step response characteristics extraction/Expected set point and step parameters ==
  Step/z : Inport
  Step : Inport  Port=2
  Static Gain : Inport  Port=3
  Trigger : TriggerPort
  Compare To Zero : simulink/Logic and Bit Operations/Compare To Zero  SystemSampleTime=-1  relop=>  LogicOutDataTypeMode=uint8  ZeroCross=off
  Divide : Product  Inputs=**  OutScaling=2^-10
  Divide1 : Product  Inputs=**  OutScaling=2^-10
  Subtract : Sum  Inputs=-+  OutScaling=2^-10
  Step sign : Outport
  Set point : Outport  Port=2
  Response step size : Outport  Port=3
  wires:
  Divide1/1 -> Response step size/1
  Compare To Zero/1 -> Step sign/1
  Subtract/1 -> Divide1/1, Compare To Zero/1
  Step/z/1 -> Subtract/1
  Step/1 -> Subtract/2, Divide/1
  Static Gain/1 -> Divide1/2, Divide/2
  Divide/1 -> Set point/1

== system MIL_Test/Validation Function/Feature extraction/Step response characteristics/Step response characteristics extraction/Extract maximum overshoot ==
  Step response : Inport
  Reset : Inport  Port=2
  Step sign : Inport  Port=3
  Active if signals constant for some specified time : Subsystem
  Detect increase : Subsystem  TreatAsAtomicUnit=on
  Detect increase1 : Subsystem  TreatAsAtomicUnit=on
  Detect increase2 : Subsystem  TreatAsAtomicUnit=on
  Hold value with counter : Subsystem  TreatAsAtomicUnit=on
  Logical Operator : Logic  Operator=OR  Inputs=3  AllPortsSameDT=off  OutDataTypeMode=Boolean
  Step response moving average and initial conditions before step : Subsystem  TreatAsAtomicUnit=on
  Subtract : Sum  Inputs=+-  OutScaling=2^-10
  Trigger hold value : Subsystem  TreatAsAtomicUnit=on
  Maximum overshoot : Outport
  wires:
  Active if signals constant for some specified time/1(Constant signals) -> Detect increase/1(Signal)
  Reset/1 -> Step response moving average and initial conditions before step/1(Reset), Hold value with counter/1(Reset counter), Detect increase2/1(Signal)
  Step sign/1 -> Trigger hold value/2(Step sign)
  Step response/1 -> Step response moving average and initial conditions before step/2(Step response), Active if signals constant for some specified time/1(Signal1), Active if signals constant for some specified time/2(Signal 2), Subtract/2, Hold value with counter/2(Value)
  Step response moving average and initial conditions before step/1(d(Step Response) average) -> Trigger hold value/1(d(Step Response) average)
  Subtract/1 -> Maximum overshoot/1
  Hold value with counter/1(Held value) -> Subtract/1
  Logical Operator/1 -> Hold value with counter/Trigger
  Detect increase/1(Increase) -> Logical Operator/1
  Detect increase2/1(Increase) -> Logical Operator/2
  Detect increase1/1(Increase) -> Logical Operator/3
  Trigger hold value/1(Overshoot Trigger) -> Detect increase1/1(Signal)

== system MIL_Test/Validation Function/Feature extraction/Step response characteristics/Step response characteristics extraction/Extract rise time ==
  Step response : Inport
  Reset : Inport  Port=2
  Set point : Inport  Port=3
  Response step size : Inport  Port=4
  100 % : Constant  Value=100
  "100% " : Constant  Value=100
  Add1 : Sum  Inputs=-+  OutScaling=2^-10
  Add2 : Sum  Inputs=+-  OutScaling=2^-10
  Clock : Clock
      settings: Decimation=10
  Divide : Product  Inputs=**/  OutScaling=2^-10
  Divide1 : Product  Inputs=**/  OutScaling=2^-10
  Logical Operator : Logic  Operator=XOR  AllPortsSameDT=off  OutDataTypeMode=Boolean
  Logical Operator1 : Logic  Operator=OR  AllPortsSameDT=off  OutDataTypeMode=Boolean
  Relational Operator : RelationalOperator  LogicOutDataTypeMode=Boolean
  Relational Operator2 : RelationalOperator  Operator=<=  LogicOutDataTypeMode=Boolean
  Time difference : Subsystem  TreatAsAtomicUnit=on
  lowerLim : Constant  Value=10
  upperLim : Constant  Value=90
  Rise time : Outport
  wires:
  Add2/1 -> Relational Operator2/2
  Response step size/1 -> Divide1/2, Divide/2
  Set point/1 -> Add2/1, Add1/2
  Add1/1 -> Relational Operator/1
  Divide/1 -> Add1/1
  100 %/1 -> Divide1/3
  "100% "/1 -> Divide/3
  Relational Operator/1 -> Logical Operator/1
  Relational Operator2/1 -> Logical Operator/2
  Divide1/1 -> Add2/2
  upperLim/1 -> Divide1/1
  lowerLim/1 -> Divide/1
  Logical Operator1/1 -> Time difference/Trigger
  Logical Operator/1 -> Logical Operator1/2
  Reset/1 -> Time difference/1(Reset counter), Logical Operator1/1
  Time difference/1(Time difference) -> Rise time/1
  Step response/1 -> Relational Operator2/1, Relational Operator/2
  Clock/1 -> Time difference/2(Clock)

== system MIL_Test/Validation Function/Feature extraction/Step response characteristics/Step response characteristics extraction/Extract settling time ==
  Step response : Inport
  Set point : Inport  Port=2
  Reset : Inport  Port=3
  Step time : Inport  Port=4
  " 100%" : Constant  Value=100
  Abs : Abs
  Abs1 : Abs
  Add : Sum  Inputs=+-  OutScaling=2^-10
  Add3 : Sum  Inputs=+-  OutScaling=2^-10
  Clock1 : Clock
      settings: Decimation=10
  Divide2 : Product  Inputs=**/  OutScaling=2^-10
  Logical Operator : Logic  Operator=OR  AllPortsSameDT=off  OutDataTypeMode=Boolean
  Logical Operator1 : Logic  Operator=NOT  AllPortsSameDT=off  OutDataTypeMode=Boolean
  Relational Operator3 : RelationalOperator  Operator=>  LogicOutDataTypeMode=Boolean
  Set point percent : Constant  Value=5
  Time stamp : Subsystem  TreatAsAtomicUnit=on
  Settling time : Outport
  wires:
  Time stamp/1(Time) -> Settling time/1
  Step time/1 -> Add/2
  Add/1 -> Time stamp/1(Clock)
  Clock1/1 -> Add/1
  Abs1/1 -> Relational Operator3/2
  Divide2/1 -> Abs1/1
  " 100%"/1 -> Divide2/3
  Abs/1 -> Relational Operator3/1
  Add3/1 -> Abs/1
  Set point percent/1 -> Divide2/2
  Step response/1 -> Add3/1
  Set point/1 -> Divide2/1, Add3/2
  Relational Operator3/1 -> Logical Operator1/1
  Logical Operator1/1 -> Logical Operator/2
  Reset/1 -> Logical Operator/1
  Logical Operator/1 -> Time stamp/Trigger
